simulink model "ValidateThrustersBLUE"  (R2020a)
settings: Solver=FixedStepAuto  StartTime=0.0  StopTime=5  RelTol=1e-3  EnableMultiTasking=on
undefined symbols (not defined in the file): Thruster1_OnTime, Thruster2_OnTime, Thruster3_OnTime, Thruster4_OnTime, Thruster5_OnTime, Thruster6_OnTime, Thruster7_OnTime, Thruster8_OnTime
libraries: raspberrypiBasiclib x10
settings Model: SimulationMode=external  ExtModeTrigDuration=2  Creator=AlexC  LastModifiedBy=SPOT
settings SolverCC: PositivePriorityOrder=on
settings DataIOCC: ReturnWorkspaceOutputs=off
settings OptimizationCC: MaxStackSize=64
settings DebuggingCC: ParameterTunabilityLossMsg=error  ArithmeticOperatorsInVariantConditions=warning
settings HardwareCC: ProdBitPerPointer=32  ProdBitPerSizeT=32  ProdBitPerPtrDiffT=32  ProdLargestAtomicInteger=Long  ProdLargestAtomicFloat=Double  ProdWordSize=32  ProdHWDeviceType=ARM Compatible->ARM Cortex  UseEmbeddedCoderFeatures=off
settings SFSimCC: SimUseLocalCustomCode=off  CustomCodeUndefinedFunction=UseInterfaceOnly
settings RTWCC: SystemTargetFile=ert.tlc  HardwareBoard=Raspberry Pi  TemplateMakefile=ert_default_tmf  GenerateReport=on  RTWUseLocalCustomCode=off  Toolchain=GNU GCC Raspberry Pi  BuildConfiguration=Faster Runs  LaunchReport=on
settings CodeAppCC: ForceParamTrailComments=on  OperatorAnnotations=on  StateflowObjectComments=on  MATLABSourceComments=on
settings ERTTargetCC: ERTCustomFileBanners=off  SupportContinuousTime=on  SupportNonInlinedSFcns=on  RemoveResetFunc=off  SupportVariableSizeSignals=on  ModelStepFunctionPrototypeControlCompliant=off

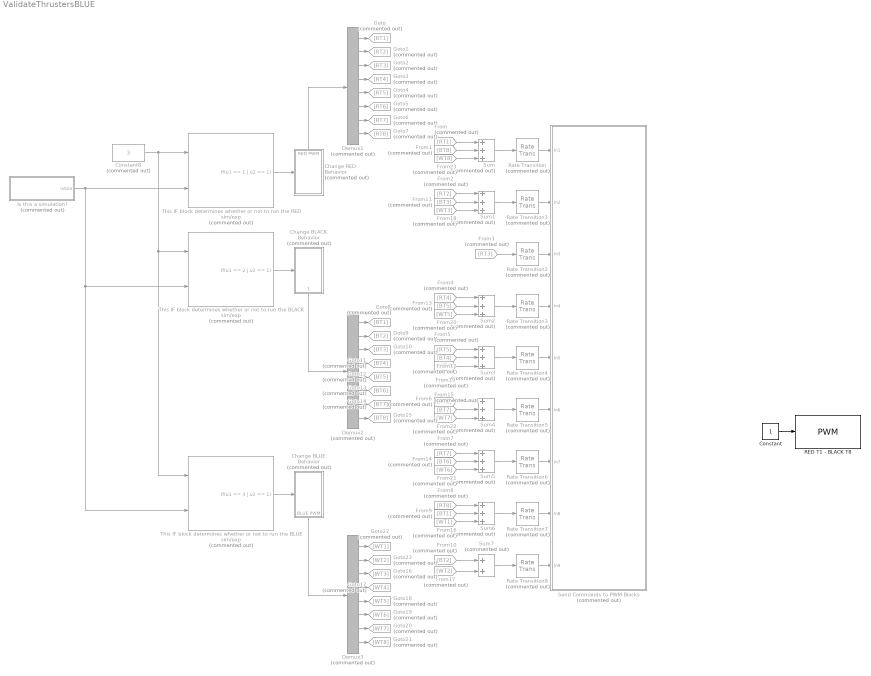
== system ValidateThrustersBLUE ==
  Change BLACK Behavior : Subsystem  Commented=on  TreatAsAtomicUnit=on
  Change BLUE Behavior : Subsystem  Commented=on  TreatAsAtomicUnit=on
  Change RED Behavior : Subsystem  Commented=on  TreatAsAtomicUnit=on
  Constant : Constant
  Constant8 : Constant  Commented=on  Value=3
  Demux1 : Demux  Commented=on  Outputs=8
  Demux2 : Demux  Commented=on  Outputs=8
  Demux3 : Demux  Commented=on  Outputs=8
  From : From  Commented=on  GotoTag=RT1
  From1 : From  Commented=on  GotoTag=BT8
  From10 : From  Commented=on  GotoTag=BT2
  From11 : From  Commented=on  GotoTag=BT3
  From12 : From  Commented=on  GotoTag=BT4
  From13 : From  Commented=on  GotoTag=BT5
  From14 : From  Commented=on  GotoTag=BT6
  From15 : From  Commented=on  GotoTag=BT7
  From16 : From  Commented=on  GotoTag=WT1
  From17 : From  Commented=on  GotoTag=WT2
  From18 : From  Commented=on  GotoTag=WT3
  From19 : From  Commented=on  GotoTag=WT4
  From2 : From  Commented=on  GotoTag=RT2
  From20 : From  Commented=on  GotoTag=WT5
  From21 : From  Commented=on  GotoTag=WT6
  From22 : From  Commented=on  GotoTag=WT7
  From23 : From  Commented=on  GotoTag=WT8
  From3 : From  Commented=on  GotoTag=RT3
  From4 : From  Commented=on  GotoTag=RT4
  From5 : From  Commented=on  GotoTag=RT5
  From6 : From  Commented=on  GotoTag=RT6
  From7 : From  Commented=on  GotoTag=RT7
  From8 : From  Commented=on  GotoTag=RT8
  From9 : From  Commented=on  GotoTag=BT1
  Goto : Goto  Commented=on  GotoTag=RT1
  Goto1 : Goto  Commented=on  GotoTag=RT2
  Goto10 : Goto  Commented=on  GotoTag=BT3
  Goto11 : Goto  Commented=on  GotoTag=BT4
  Goto12 : Goto  Commented=on  GotoTag=BT5
  Goto13 : Goto  Commented=on  GotoTag=BT6
  Goto14 : Goto  Commented=on  GotoTag=BT7
  Goto15 : Goto  Commented=on  GotoTag=BT8
  Goto16 : Goto  Commented=on  GotoTag=WT3
  Goto17 : Goto  Commented=on  GotoTag=WT4
  Goto18 : Goto  Commented=on  GotoTag=WT5
  Goto19 : Goto  Commented=on  GotoTag=WT6
  Goto2 : Goto  Commented=on  GotoTag=RT3
  Goto20 : Goto  Commented=on  GotoTag=WT7
  Goto21 : Goto  Commented=on  GotoTag=WT8
  Goto22 : Goto  Commented=on  GotoTag=WT1
  Goto23 : Goto  Commented=on  GotoTag=WT2
  Goto3 : Goto  Commented=on  GotoTag=RT4
  Goto4 : Goto  Commented=on  GotoTag=RT5
  Goto5 : Goto  Commented=on  GotoTag=RT6
  Goto6 : Goto  Commented=on  GotoTag=RT7
  Goto7 : Goto  Commented=on  GotoTag=RT8
  Goto8 : Goto  Commented=on  GotoTag=BT1
  Goto9 : Goto  Commented=on  GotoTag=BT2
  Is this a simulation? : Subsystem  Commented=on
  RED T1 - BLACK T8 : raspberrypiBasiclib/PWM  board=Pi 3 Model B  Pin_=17  Frequency=10  blockPlatform=Raspberry Pi
      settings: SourceProductBaseCode=RASPPI
  Rate Transition{,1..8} (9 alike) : RateTransition  Commented=on  OutPortSampleTime=0.1
  Send Commands to PWM Blocks : Subsystem  Commented=on  TreatAsAtomicUnit=on  SystemSampleTime=0.1
  Sum{,1..6} (7 alike) : Sum  Commented=on  Inputs=+++
  Sum7 : Sum  Commented=on
  This IF block determines whether or not to run the BLACK sim/exp : If  Commented=on  NumInputs=2  IfExpression=u1 == 2 | u2 == 1  ShowElse=off
  This IF block determines whether or not to run the BLUE sim/exp : If  Commented=on  NumInputs=2  IfExpression=u1 == 3 | u2 == 1  ShowElse=off
  "This IF block determines whether or not to run the RED sim/exp " : If  Commented=on  NumInputs=2  IfExpression=u1 == 1 | u2 == 1  ShowElse=off
  wires:
  Demux3/8 -> Goto21/1
  Rate Transition2/1 -> Send Commands to PWM Blocks/3(In3)
  Sum6/1 -> Rate Transition7/1
  This IF block determines whether or not to run the BLUE sim/exp/1 -> Change BLUE Behavior/Action
  Demux2/2 -> Goto9/1
  This IF block determines whether or not to run the BLACK sim/exp/1 -> Change BLACK Behavior/Action
  Constant8/1 -> This IF block determines whether or not to run the BLUE sim/exp/1, This IF block determines whether or not to run the BLACK sim/exp/1, "This IF block determines whether or not to run the RED sim/exp "/1
  Demux2/4 -> Goto11/1
  Rate Transition5/1 -> Send Commands to PWM Blocks/6(In6)
  Demux3/4 -> Goto17/1
  Rate Transition8/1 -> Send Commands to PWM Blocks/9(In9)
  Demux3/7 -> Goto20/1
  From4/1 -> Sum2/1
  Rate Transition7/1 -> Send Commands to PWM Blocks/8(In8)
  Sum4/1 -> Rate Transition5/1
  Demux1/7 -> Goto6/1
  Demux3/6 -> Goto19/1
  Demux1/8 -> Goto7/1
  Demux1/3 -> Goto2/1
  Sum3/1 -> Rate Transition4/1
  Sum5/1 -> Rate Transition6/1
  Sum2/1 -> Rate Transition3/1
  Change RED Behavior/1(RED PWM) -> Demux1/1
  From13/1 -> Sum2/2
  From15/1 -> Sum4/2
  From11/1 -> Sum1/2
  From2/1 -> Sum1/1
  From14/1 -> Sum5/2
  From1/1 -> Sum/2
  From7/1 -> Sum5/1
  Rate Transition3/1 -> Send Commands to PWM Blocks/4(In4)
  Change BLACK Behavior/1(BLACK PWM) -> Demux2/1
  Demux2/3 -> Goto10/1
  Demux2/6 -> Goto13/1
  Demux1/6 -> Goto5/1
  From9/1 -> Sum6/2
  Demux2/7 -> Goto14/1
  Demux1/4 -> Goto3/1
  Is this a simulation?/1(isSim) -> This IF block determines whether or not to run the BLACK sim/exp/2, This IF block determines whether or not to run the BLUE sim/exp/2, "This IF block determines whether or not to run the RED sim/exp "/2
  Rate Transition4/1 -> Send Commands to PWM Blocks/5(In5)
  Demux2/5 -> Goto12/1
  From18/1 -> Sum1/3
  Demux3/5 -> Goto18/1
  Demux1/2 -> Goto1/1
  From/1 -> Sum/1
  From16/1 -> Sum6/3
  Demux3/3 -> Goto16/1
  Sum/1 -> Rate Transition/1
  Sum7/1 -> Rate Transition8/1
  Demux2/8 -> Goto15/1
  From8/1 -> Sum6/1
  From12/1 -> Sum3/2
  Change BLUE Behavior/1(BLUE PWM) -> Demux3/1
  Rate Transition6/1 -> Send Commands to PWM Blocks/7(In7)
  Demux1/5 -> Goto4/1
  From5/1 -> Sum3/1
  Demux3/1 -> Goto22/1
  Demux2/1 -> Goto8/1
  From21/1 -> Sum5/3
  From17/1 -> Sum7/2
  "This IF block determines whether or not to run the RED sim/exp "/1 -> Change RED Behavior/Action
  From22/1 -> Sum4/3
  From6/1 -> Sum4/1
  From20/1 -> Sum2/3
  Sum1/1 -> Rate Transition1/1
  Demux3/2 -> Goto23/1
  From10/1 -> Sum7/1
  From19/1 -> Sum3/3
  Demux1/1 -> Goto/1
  Rate Transition/1 -> Send Commands to PWM Blocks/1(In1)
  From23/1 -> Sum/3
  From3/1 -> Rate Transition2/1
  Rate Transition1/1 -> Send Commands to PWM Blocks/2(In2)
  Constant/1 -> RED T1 - BLACK T8/1

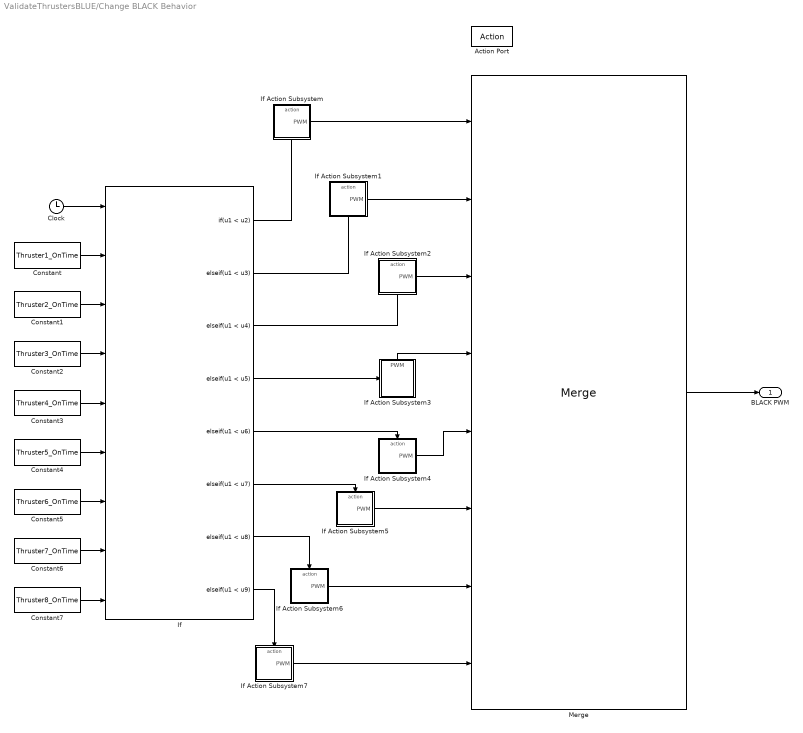
== system ValidateThrustersBLUE/Change BLACK Behavior ==
  Action Port : ActionPort  ActionPortLabel=if(u1 == 2 | u2 == 1)
  Clock : Clock
  Constant : Constant  Value=Thruster1_OnTime
  Constant1 : Constant  Value=Thruster2_OnTime
  Constant2 : Constant  Value=Thruster3_OnTime
  Constant3 : Constant  Value=Thruster4_OnTime
  Constant4 : Constant  Value=Thruster5_OnTime
  Constant5 : Constant  Value=Thruster6_OnTime
  Constant6 : Constant  Value=Thruster7_OnTime
  Constant7 : Constant  Value=Thruster8_OnTime
  If : If  NumInputs=9  IfExpression=u1 < u2  ElseIfExpressions=u1 < u3, u1 < u4, u1 < u5, u1 < u6, u1 < u7, u1 < u8, u1 < u9  ShowElse=off
  If Action Subsystem : Subsystem  TreatAsAtomicUnit=on
  If Action Subsystem1 : Subsystem  TreatAsAtomicUnit=on
  If Action Subsystem2 : Subsystem  TreatAsAtomicUnit=on
  If Action Subsystem3 : Subsystem  TreatAsAtomicUnit=on
  If Action Subsystem5 : Subsystem  TreatAsAtomicUnit=on
  If Action Subsystem6 : Subsystem  TreatAsAtomicUnit=on
  If Action Subsystem7 : Subsystem  TreatAsAtomicUnit=on
  If Action Subsystem4 : Subsystem  TreatAsAtomicUnit=on
  Merge : Merge  Inputs=8
  BLACK PWM : Outport  VectorParamsAs1DForOutWhenUnconnected=off
  wires:
  Merge/1 -> BLACK PWM/1
  If/7 -> If Action Subsystem6/Action
  Constant6/1 -> If/8
  If/3 -> If Action Subsystem2/Action
  Constant4/1 -> If/6
  Constant3/1 -> If/5
  If Action Subsystem1/1(PWM) -> Merge/2
  If Action Subsystem2/1(PWM) -> Merge/3
  Constant/1 -> If/2
  Constant5/1 -> If/7
  Constant2/1 -> If/4
  If/5 -> If Action Subsystem4/Action
  If/6 -> If Action Subsystem5/Action
  If/8 -> If Action Subsystem7/Action
  Constant7/1 -> If/9
  If/2 -> If Action Subsystem1/Action
  If Action Subsystem4/1(PWM) -> Merge/5
  If Action Subsystem5/1(PWM) -> Merge/6
  If/4 -> If Action Subsystem3/Action
  If Action Subsystem/1(PWM) -> Merge/1
  If/1 -> If Action Subsystem/Action
  Clock/1 -> If/1
  Constant1/1 -> If/3
  If Action Subsystem6/1(PWM) -> Merge/7
  If Action Subsystem7/1(PWM) -> Merge/8
  If Action Subsystem3/1(PWM) -> Merge/4

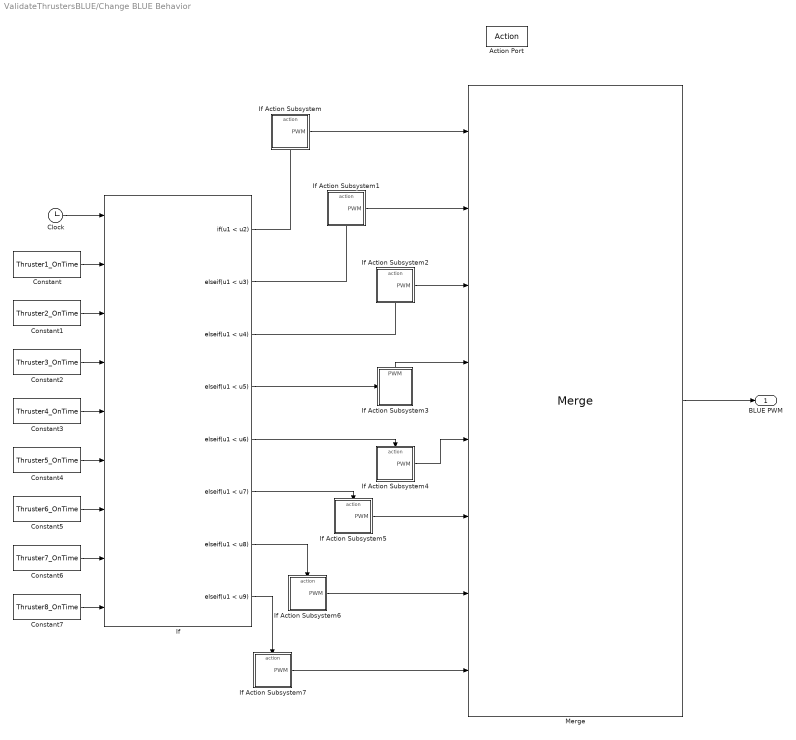
== system ValidateThrustersBLUE/Change BLUE Behavior ==
  Action Port : ActionPort  ActionPortLabel=if(u1 == 3 | u2 == 1)
  Clock : Clock
  Constant : Constant  Value=Thruster1_OnTime
  Constant1 : Constant  Value=Thruster2_OnTime
  Constant2 : Constant  Value=Thruster3_OnTime
  Constant3 : Constant  Value=Thruster4_OnTime
  Constant4 : Constant  Value=Thruster5_OnTime
  Constant5 : Constant  Value=Thruster6_OnTime
  Constant6 : Constant  Value=Thruster7_OnTime
  Constant7 : Constant  Value=Thruster8_OnTime
  If : If  NumInputs=9  IfExpression=u1 < u2  ElseIfExpressions=u1 < u3, u1 < u4, u1 < u5, u1 < u6, u1 < u7, u1 < u8, u1 < u9  ShowElse=off
  If Action Subsystem : Subsystem  TreatAsAtomicUnit=on
  If Action Subsystem1 : Subsystem  TreatAsAtomicUnit=on
  If Action Subsystem2 : Subsystem  TreatAsAtomicUnit=on
  If Action Subsystem3 : Subsystem  TreatAsAtomicUnit=on
  If Action Subsystem5 : Subsystem  TreatAsAtomicUnit=on
  If Action Subsystem6 : Subsystem  TreatAsAtomicUnit=on
  If Action Subsystem7 : Subsystem  TreatAsAtomicUnit=on
  If Action Subsystem4 : Subsystem  TreatAsAtomicUnit=on
  Merge : Merge  Inputs=8
  BLUE PWM : Outport  VectorParamsAs1DForOutWhenUnconnected=off
  wires:
  Merge/1 -> BLUE PWM/1
  If/7 -> If Action Subsystem6/Action
  Constant6/1 -> If/8
  If/3 -> If Action Subsystem2/Action
  Constant4/1 -> If/6
  Constant3/1 -> If/5
  If Action Subsystem1/1(PWM) -> Merge/2
  If Action Subsystem2/1(PWM) -> Merge/3
  Constant/1 -> If/2
  Constant5/1 -> If/7
  Constant2/1 -> If/4
  If/5 -> If Action Subsystem4/Action
  If/6 -> If Action Subsystem5/Action
  If/8 -> If Action Subsystem7/Action
  Constant7/1 -> If/9
  If/2 -> If Action Subsystem1/Action
  If Action Subsystem4/1(PWM) -> Merge/5
  If Action Subsystem5/1(PWM) -> Merge/6
  If/4 -> If Action Subsystem3/Action
  If Action Subsystem/1(PWM) -> Merge/1
  If/1 -> If Action Subsystem/Action
  Clock/1 -> If/1
  Constant1/1 -> If/3
  If Action Subsystem6/1(PWM) -> Merge/7
  If Action Subsystem7/1(PWM) -> Merge/8
  If Action Subsystem3/1(PWM) -> Merge/4

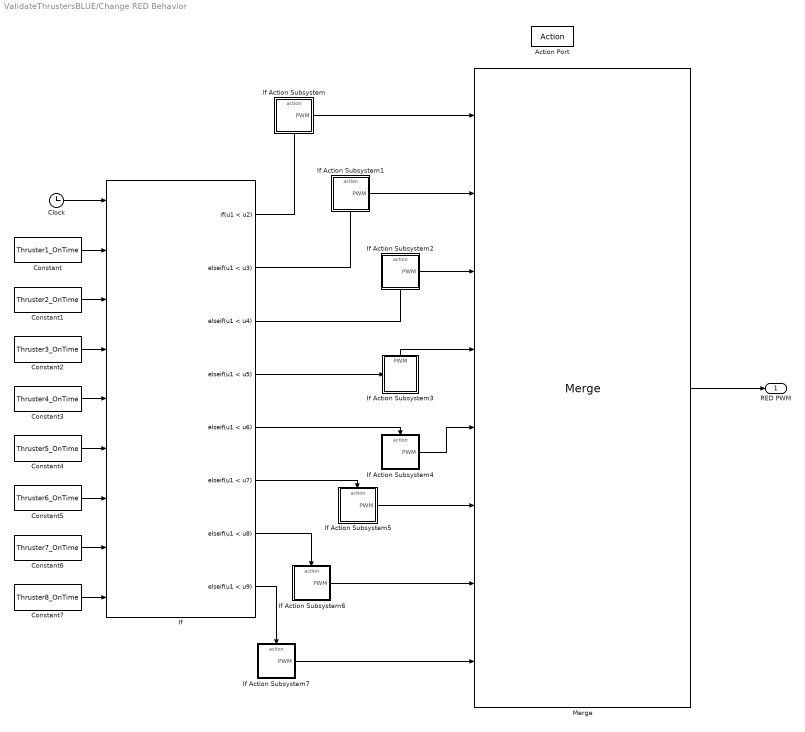
== system ValidateThrustersBLUE/Change RED Behavior ==
  Action Port : ActionPort  ActionPortLabel=if(u1 == 1 | u2 == 1)
  Clock : Clock
  Constant : Constant  Value=Thruster1_OnTime
  Constant1 : Constant  Value=Thruster2_OnTime
  Constant2 : Constant  Value=Thruster3_OnTime
  Constant3 : Constant  Value=Thruster4_OnTime
  Constant4 : Constant  Value=Thruster5_OnTime
  Constant5 : Constant  Value=Thruster6_OnTime
  Constant6 : Constant  Value=Thruster7_OnTime
  Constant7 : Constant  Value=Thruster8_OnTime
  If : If  NumInputs=9  IfExpression=u1 < u2  ElseIfExpressions=u1 < u3, u1 < u4, u1 < u5, u1 < u6, u1 < u7, u1 < u8, u1 < u9  ShowElse=off
  If Action Subsystem : Subsystem  TreatAsAtomicUnit=on
  If Action Subsystem1 : Subsystem  TreatAsAtomicUnit=on
  If Action Subsystem2 : Subsystem  TreatAsAtomicUnit=on
  If Action Subsystem3 : Subsystem  TreatAsAtomicUnit=on
  If Action Subsystem5 : Subsystem  TreatAsAtomicUnit=on
  If Action Subsystem6 : Subsystem  TreatAsAtomicUnit=on
  If Action Subsystem7 : Subsystem  TreatAsAtomicUnit=on
  If Action Subsystem4 : Subsystem  TreatAsAtomicUnit=on
  Merge : Merge  Inputs=8
  RED PWM : Outport  VectorParamsAs1DForOutWhenUnconnected=off
  wires:
  Merge/1 -> RED PWM/1
  If/7 -> If Action Subsystem6/Action
  If Action Subsystem7/1(PWM) -> Merge/8
  If Action Subsystem3/1(PWM) -> Merge/4
  Constant1/1 -> If/3
  If Action Subsystem6/1(PWM) -> Merge/7
  Clock/1 -> If/1
  If/1 -> If Action Subsystem/Action
  If Action Subsystem4/1(PWM) -> Merge/5
  If Action Subsystem5/1(PWM) -> Merge/6
  If/4 -> If Action Subsystem3/Action
  If Action Subsystem/1(PWM) -> Merge/1
  Constant7/1 -> If/9
  If/6 -> If Action Subsystem5/Action
  If/5 -> If Action Subsystem4/Action
  If/8 -> If Action Subsystem7/Action
  Constant2/1 -> If/4
  Constant5/1 -> If/7
  Constant/1 -> If/2
  If Action Subsystem2/1(PWM) -> Merge/3
  If/2 -> If Action Subsystem1/Action
  If Action Subsystem1/1(PWM) -> Merge/2
  Constant3/1 -> If/5
  Constant4/1 -> If/6
  If/3 -> If Action Subsystem2/Action
  Constant6/1 -> If/8

== system ValidateThrustersBLUE/Is this a simulation? ==
  Constant : Constant  SampleTime=-1
  isSim : Outport  VectorParamsAs1DForOutWhenUnconnected=off
  wires:
  Constant/1 -> isSim/1

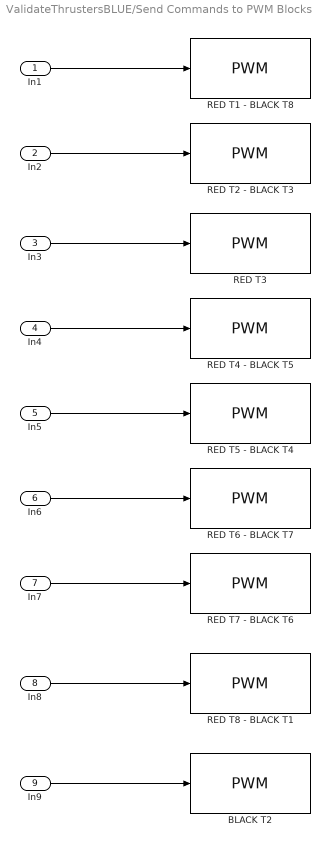
== system ValidateThrustersBLUE/Send Commands to PWM Blocks ==
  In1 : Inport
  In2 : Inport  Port=2
  In3 : Inport  Port=3
  In4 : Inport  Port=4
  In5 : Inport  Port=5
  In6 : Inport  Port=6
  In7 : Inport  Port=7
  In8 : Inport  Port=8
  In9 : Inport  Port=9
  BLACK T2 : raspberrypiBasiclib/PWM  board=Pi 3 Model B  Pin_=9  Frequency=10  blockPlatform=Raspberry Pi
      settings: SourceProductBaseCode=RASPPI
  RED T1 - BLACK T8 : raspberrypiBasiclib/PWM  board=Pi 3 Model B  Pin_=27  Frequency=10  blockPlatform=Raspberry Pi
      settings: SourceProductBaseCode=RASPPI
  RED T2 - BLACK T3 : raspberrypiBasiclib/PWM  board=Pi 3 Model B  Pin_=19  Frequency=10  blockPlatform=Raspberry Pi
      settings: SourceProductBaseCode=RASPPI
  RED T3 : raspberrypiBasiclib/PWM  board=Pi 3 Model B  Pin_=4  Frequency=10  blockPlatform=Raspberry Pi
      settings: SourceProductBaseCode=RASPPI
  RED T4 - BLACK T5 : raspberrypiBasiclib/PWM  board=Pi 3 Model B  Pin_=22  Frequency=10  blockPlatform=Raspberry Pi
      settings: SourceProductBaseCode=RASPPI
  RED T5 - BLACK T4 : raspberrypiBasiclib/PWM  board=Pi 3 Model B  Pin_=5  Frequency=10  blockPlatform=Raspberry Pi
      settings: SourceProductBaseCode=RASPPI
  RED T6 - BLACK T7 : raspberrypiBasiclib/PWM  board=Pi 3 Model B  Pin_=6  Frequency=10  blockPlatform=Raspberry Pi
      settings: SourceProductBaseCode=RASPPI
  RED T7 - BLACK T6 : raspberrypiBasiclib/PWM  board=Pi 3 Model B  Pin_=13  Frequency=10  blockPlatform=Raspberry Pi
      settings: SourceProductBaseCode=RASPPI
  RED T8 - BLACK T1 : raspberrypiBasiclib/PWM  board=Pi 3 Model B  Pin_=17  Frequency=10  blockPlatform=Raspberry Pi
      settings: SourceProductBaseCode=RASPPI
  wires:
  In4/1 -> RED T4 - BLACK T5/1
  In5/1 -> RED T5 - BLACK T4/1
  In1/1 -> RED T1 - BLACK T8/1
  In8/1 -> RED T8 - BLACK T1/1
  In9/1 -> BLACK T2/1
  In7/1 -> RED T7 - BLACK T6/1
  In6/1 -> RED T6 - BLACK T7/1
  In3/1 -> RED T3/1
  In2/1 -> RED T2 - BLACK T3/1

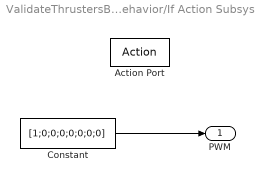
== system ValidateThrustersBLUE/Change BLACK Behavior/If Action Subsystem ==
  Action Port : ActionPort  ActionPortLabel=if(u1 < u2)
  Constant : Constant  Value=[1;0;0;0;0;0;0;0]
  PWM : Outport  VectorParamsAs1DForOutWhenUnconnected=off
  wires:
  Constant/1 -> PWM/1

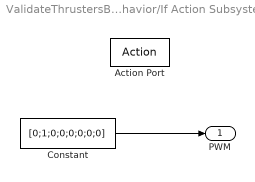
== system ValidateThrustersBLUE/Change BLACK Behavior/If Action Subsystem1 ==
  Action Port : ActionPort  ActionPortLabel=elseif(u1 < u3)
  Constant : Constant  Value=[0;1;0;0;0;0;0;0]
  PWM : Outport  VectorParamsAs1DForOutWhenUnconnected=off
  wires:
  Constant/1 -> PWM/1

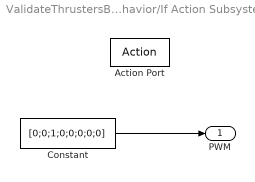
== system ValidateThrustersBLUE/Change BLACK Behavior/If Action Subsystem2 ==
  Action Port : ActionPort  ActionPortLabel=elseif( u1 < u4)
  Constant : Constant  Value=[0;0;1;0;0;0;0;0]
  PWM : Outport  VectorParamsAs1DForOutWhenUnconnected=off
  wires:
  Constant/1 -> PWM/1

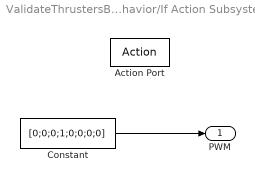
== system ValidateThrustersBLUE/Change BLACK Behavior/If Action Subsystem3 ==
  Action Port : ActionPort  ActionPortLabel=elseif( u1 < u5)
  Constant : Constant  Value=[0;0;0;1;0;0;0;0]
  PWM : Outport  VectorParamsAs1DForOutWhenUnconnected=off
  wires:
  Constant/1 -> PWM/1

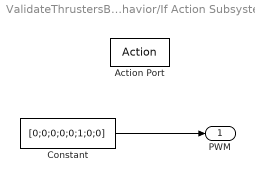
== system ValidateThrustersBLUE/Change BLACK Behavior/If Action Subsystem5 ==
  Action Port : ActionPort  ActionPortLabel=elseif( u1 < u7)
  Constant : Constant  Value=[0;0;0;0;0;1;0;0]
  PWM : Outport  VectorParamsAs1DForOutWhenUnconnected=off
  wires:
  Constant/1 -> PWM/1

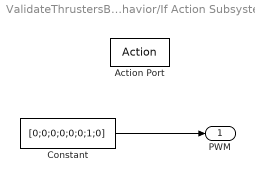
== system ValidateThrustersBLUE/Change BLACK Behavior/If Action Subsystem6 ==
  Action Port : ActionPort  ActionPortLabel=elseif( u1 < u8)
  Constant : Constant  Value=[0;0;0;0;0;0;1;0]
  PWM : Outport  VectorParamsAs1DForOutWhenUnconnected=off
  wires:
  Constant/1 -> PWM/1

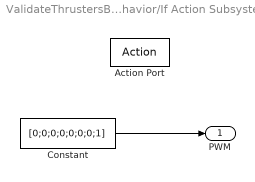
== system ValidateThrustersBLUE/Change BLACK Behavior/If Action Subsystem7 ==
  Action Port : ActionPort  ActionPortLabel=elseif( u1 < u9)
  Constant : Constant  Value=[0;0;0;0;0;0;0;1]
  PWM : Outport  VectorParamsAs1DForOutWhenUnconnected=off
  wires:
  Constant/1 -> PWM/1

== system ValidateThrustersBLUE/Change BLACK Behavior/If Action Subsystem4 ==
  Action Port : ActionPort  ActionPortLabel=elseif( u1 < u6)
  Constant : Constant  Value=[0;0;0;0;1;0;0;0]
  PWM : Outport  VectorParamsAs1DForOutWhenUnconnected=off
  wires:
  Constant/1 -> PWM/1

== system ValidateThrustersBLUE/Change BLUE Behavior/If Action Subsystem ==
  Action Port : ActionPort  ActionPortLabel=if(u1 < u2)
  Constant : Constant  Value=[1;0;0;0;0;0;0;0]
  PWM : Outport  VectorParamsAs1DForOutWhenUnconnected=off
  wires:
  Constant/1 -> PWM/1

== system ValidateThrustersBLUE/Change BLUE Behavior/If Action Subsystem1 ==
  Action Port : ActionPort  ActionPortLabel=elseif(u1 < u3)
  Constant : Constant  Value=[0;1;0;0;0;0;0;0]
  PWM : Outport  VectorParamsAs1DForOutWhenUnconnected=off
  wires:
  Constant/1 -> PWM/1

== system ValidateThrustersBLUE/Change BLUE Behavior/If Action Subsystem2 ==
  Action Port : ActionPort  ActionPortLabel=elseif( u1 < u4)
  Constant : Constant  Value=[0;0;1;0;0;0;0;0]
  PWM : Outport  VectorParamsAs1DForOutWhenUnconnected=off
  wires:
  Constant/1 -> PWM/1

== system ValidateThrustersBLUE/Change BLUE Behavior/If Action Subsystem3 ==
  Action Port : ActionPort  ActionPortLabel=elseif( u1 < u5)
  Constant : Constant  Value=[0;0;0;1;0;0;0;0]
  PWM : Outport  VectorParamsAs1DForOutWhenUnconnected=off
  wires:
  Constant/1 -> PWM/1

== system ValidateThrustersBLUE/Change BLUE Behavior/If Action Subsystem5 ==
  Action Port : ActionPort  ActionPortLabel=elseif( u1 < u7)
  Constant : Constant  Value=[0;0;0;0;0;1;0;0]
  PWM : Outport  VectorParamsAs1DForOutWhenUnconnected=off
  wires:
  Constant/1 -> PWM/1

== system ValidateThrustersBLUE/Change BLUE Behavior/If Action Subsystem6 ==
  Action Port : ActionPort  ActionPortLabel=elseif( u1 < u8)
  Constant : Constant  Value=[0;0;0;0;0;0;1;0]
  PWM : Outport  VectorParamsAs1DForOutWhenUnconnected=off
  wires:
  Constant/1 -> PWM/1

== system ValidateThrustersBLUE/Change BLUE Behavior/If Action Subsystem7 ==
  Action Port : ActionPort  ActionPortLabel=elseif( u1 < u9)
  Constant : Constant  Value=[0;0;0;0;0;0;0;1]
  PWM : Outport  VectorParamsAs1DForOutWhenUnconnected=off
  wires:
  Constant/1 -> PWM/1

== system ValidateThrustersBLUE/Change BLUE Behavior/If Action Subsystem4 ==
  Action Port : ActionPort  ActionPortLabel=elseif( u1 < u6)
  Constant : Constant  Value=[0;0;0;0;1;0;0;0]
  PWM : Outport  VectorParamsAs1DForOutWhenUnconnected=off
  wires:
  Constant/1 -> PWM/1

== system ValidateThrustersBLUE/Change RED Behavior/If Action Subsystem ==
  Action Port : ActionPort  ActionPortLabel=if(u1 < u2)
  Constant : Constant  Value=[1;0;0;0;0;0;0;0]
  PWM : Outport  VectorParamsAs1DForOutWhenUnconnected=off
  wires:
  Constant/1 -> PWM/1

== system ValidateThrustersBLUE/Change RED Behavior/If Action Subsystem1 ==
  Action Port : ActionPort  ActionPortLabel=elseif(u1 < u3)
  Constant : Constant  Value=[0;1;0;0;0;0;0;0]
  PWM : Outport  VectorParamsAs1DForOutWhenUnconnected=off
  wires:
  Constant/1 -> PWM/1

== system ValidateThrustersBLUE/Change RED Behavior/If Action Subsystem2 ==
  Action Port : ActionPort  ActionPortLabel=elseif( u1 < u4)
  Constant : Constant  Value=[0;0;1;0;0;0;0;0]
  PWM : Outport  VectorParamsAs1DForOutWhenUnconnected=off
  wires:
  Constant/1 -> PWM/1

== system ValidateThrustersBLUE/Change RED Behavior/If Action Subsystem3 ==
  Action Port : ActionPort  ActionPortLabel=elseif( u1 < u5)
  Constant : Constant  Value=[0;0;0;1;0;0;0;0]
  PWM : Outport  VectorParamsAs1DForOutWhenUnconnected=off
  wires:
  Constant/1 -> PWM/1

== system ValidateThrustersBLUE/Change RED Behavior/If Action Subsystem5 ==
  Action Port : ActionPort  ActionPortLabel=elseif( u1 < u7)
  Constant : Constant  Value=[0;0;0;0;0;1;0;0]
  PWM : Outport  VectorParamsAs1DForOutWhenUnconnected=off
  wires:
  Constant/1 -> PWM/1

== system ValidateThrustersBLUE/Change RED Behavior/If Action Subsystem6 ==
  Action Port : ActionPort  ActionPortLabel=elseif( u1 < u8)
  Constant : Constant  Value=[0;0;0;0;0;0;1;0]
  PWM : Outport  VectorParamsAs1DForOutWhenUnconnected=off
  wires:
  Constant/1 -> PWM/1

== system ValidateThrustersBLUE/Change RED Behavior/If Action Subsystem7 ==
  Action Port : ActionPort  ActionPortLabel=elseif( u1 < u9)
  Constant : Constant  Value=[0;0;0;0;0;0;0;1]
  PWM : Outport  VectorParamsAs1DForOutWhenUnconnected=off
  wires:
  Constant/1 -> PWM/1

== system ValidateThrustersBLUE/Change RED Behavior/If Action Subsystem4 ==
  Action Port : ActionPort  ActionPortLabel=elseif( u1 < u6)
  Constant : Constant  Value=[0;0;0;0;1;0;0;0]
  PWM : Outport  VectorParamsAs1DForOutWhenUnconnected=off
  wires:
  Constant/1 -> PWM/1
